simulink model "HvCoorn"  (R2022b)
settings: configuration reference "Icar05FusaMdlCfg" (kept outside this file)
undefined symbols (not defined in the file): BMSActSt_ACChrg, BMSActSt_DCChrg, BMSActSt_disconnect, BMSActSt_offline, BMSActSt_online, BMSActSt_undefined, BMSMainNegRlySt_Clsd_SC, BMSMainNegRlySt_Open_SC, BMSMainNegRlySt_StuckInClsd_SC, BMSMainNegRlySt_StuckInOpen_SC, BMSMainPosRlySt_Clsd_SC, BMSMainPosRlySt_Open_SC, BMSMainPosRlySt_StuckInClsd_SC, BMSPrecRlySt_StuckInOpen_SC, BMSReqSt_ACChrg, BMSReqSt_DCChrg, BMSReqSt_emergencyOffline, BMSReqSt_offline, BMSReqSt_online, Chrg_stCycleBookMod_SC, Chrg_stSingleBookMod_SC, CmpgMod_stInactv_SC, DCDCActSt_buck, DCDCActSt_connected, DCDCActSt_disconnected, DCDCReqSt_buck, DCDCReqSt_standby, EngStrtStop_RefuModDft_SC, EPBActSt_Appld_SC, GearLvr_stDrvGearD_SC, GearLvr_stDrvGearN_SC, GearLvr_stDrvGearP_SC, GearLvr_stDrvGearR_SC, hpp_bACChargeLinkIni_C, hpp_bACChargeLinkOKIni_C, hpp_bAcChgEnaIni_C, hpp_bAcChgPauseIni_C, hpp_bAcLinkTempErrIni_C, hpp_bBattWarmReqIni_C, hpp_bHvilHwErrIni_C, hpp_bHvilStOkIni_C, hpp_bHvRelayClsActIni_C, hpp_bHvRelayOpnActIni_C, hpp_bHvRelayStuckIni_C, hpp_bParked4ChDchgIni_C, hpp_bRemLvBatMntnReqIni_C, hpp_bStartUpReqIni_C, hpp_stHvilCanIni_C, hpp_stWarmTimeCfgRespIni_C, HvCoorn_bAuthEnaSwt_C, HvCoorn_bAuthFailSpdLimOvrd_C, HvCoorn_bAuthFailSpdLimOvrdVal_C, HvCoorn_bAuthStrt_C, HvCoorn_bBMSUnexpdDcnctFailEna_C, HvCoorn_bBuck2RdyBypDCDCEna_C, HvCoorn_bDCChrgFctCfg_C, HvCoorn_bDcChrgWkupEnaChrgLink_C, HvCoorn_bDCDcnct4ACEna_C, HvCoorn_bDCNotBuck2ShtdwnEna_C, HvCoorn_bDrvrLevNotRdyEna_C ... (+295)
libraries: ITKLib x213, simulink x61
(part 9 of 12)

== system HvCoorn/HvCoorn/HVP_HighVoltagePowerOnOffProcedure/A01_HighvoltPowerUpReq/B01_HvRelayClsAct ==
  note: This subsystem calculates the actual status of Hv relay, for example closed, open, stuck, based on the actual status of Hv battery, the main positive relay, the main negative relay, and the precharge relay.
  note: Documentation
  icbms_stMainPosRly : Inport
  icbms_stPrecRly : Inport  Port=2
  icbms_stMainNegRly : Inport  Port=3
  icbms_stHvBat : Inport  Port=4
  Copyright : simulink/Model-Wide Utilities/Model Info  Frame=on  DisplayStringWithTags=|  HorizontalTextAlignment=Left  LeftAlignmentValue=0.02
      | © ITK Engineering Technology (Wu Xi) Co., Ltd. (ITKC)
      | 
      | Model Version: %<ModelVersion>
      | Date: %<LastModificationDate>
  InlineDescription : ITKLib/Special/InlineDescription  Tag=HideFromReport  Description=高压继电器状态确认  ShowInLibBrowser=0  RefreshPar=0
      settings: SourceProductName=ITKC_Lib
  Logical Operator1 : Logic  Operator=OR  Inputs=3  AllPortsSameDT=off  OutDataTypeStr=boolean
  Logical Operator2 : Logic  Operator=OR  Inputs=3  AllPortsSameDT=off  OutDataTypeStr=boolean
  Logical Operator3 : Logic  Operator=OR  AllPortsSameDT=off  OutDataTypeStr=boolean
  Logical Operator4 : Logic  AllPortsSameDT=off  OutDataTypeStr=boolean
  Logical Operator5 : Logic  Operator=OR  AllPortsSameDT=off  OutDataTypeStr=boolean
  Logical Operator6 : Logic  AllPortsSameDT=off  OutDataTypeStr=boolean
  Logical Operator7 : Logic  Operator=OR  AllPortsSameDT=off  OutDataTypeStr=boolean
  Relational Operator{1..13} (13 alike) : RelationalOperator  Operator===  OutDataTypeStr=boolean  InputSameDT=off
  Switch : Switch  Criteria=u2 ~= 0  SaturateOnIntegerOverflow=off  InputSameDT=off
      settings: AttributesFormatString=Criteria : %<Criteria>
  Unit detailed design : simulink/Model-Wide Utilities/DocBlock  Tag=HideFromReport  DocumentType=Text
      content=|
      | SMiVCU-3250 - 高压继电器闭合标志位
      | <电池状态>为0x4:online，或0x9：ACChrg，或0x8：DCChrg，则认为当前高压继电器为闭合状态，激活[高压继电器闭合标志位]。
      |
      | SMiVCU-3251 - 高压继电器断开标志位
      | <电池状态>为0x1：offline，或0x0：undefined，或<主正继电器状态>为0x1：open，或<主负继电器状态>为0x1：open，则认为当前高压继电器为断开状态，激活[高压继电器断开标志位]。
      |
      | SMiVCU-3252 - 高压继电器粘连标志位
      | 同时满足以下条件，则激活[高压继电器粘连标志位]
      | 1.<主正继电器状态>为0x4：StucInClsd或<预充继电器状态>为0x3：StucInOpen；
      | 2.<主负继电器状态>为0x4：StucInClsd或0x3：StucInOpen；
  hpp_tiHvilOkDelay_C : Constant  Description=[0]  Value=HvCoorn_bHvRlyClsJudgByMod_C
      settings: AttributesFormatString=%<Description>
  icbms_acCharge : Constant  Description=[9]  Value=BMSActSt_ACChrg  OutDataTypeStr=uint8
      settings: AttributesFormatString=[9]
  icbms_dcCharge : Constant  Description=[8]  Value=BMSActSt_DCChrg  OutDataTypeStr=uint8
      settings: AttributesFormatString=[8]
  icbms_offline : Constant  Description=[1]  Value=BMSActSt_offline  OutDataTypeStr=uint8
      settings: AttributesFormatString=[1]
  icbms_online : Constant  Description=[4]  Value=BMSActSt_online  OutDataTypeStr=uint8
      settings: AttributesFormatString=[4]
  icbms_undefined : Constant  Description=[0]  Value=BMSActSt_undefined  OutDataTypeStr=uint8
      settings: AttributesFormatString=[0]
  icbms_undefined1 : Constant  Description=[4]  Value=BMSMainPosRlySt_StuckInClsd_SC  OutDataTypeStr=uint8
      settings: AttributesFormatString=%<Description>
  icbms_undefined2 : Constant  Description=[4]  Value=BMSMainNegRlySt_StuckInClsd_SC  OutDataTypeStr=uint8
      settings: AttributesFormatString=%<Description>
  icbms_undefined3 : Constant  Description=[3]  Value=BMSMainNegRlySt_StuckInOpen_SC  OutDataTypeStr=uint8
      settings: AttributesFormatString=%<Description>
  icbms_undefined4 : Constant  Description=[3]  Value=BMSPrecRlySt_StuckInOpen_SC  OutDataTypeStr=uint8
      settings: AttributesFormatString=%<Description>
  icbms_undefined5 : Constant  Description=[2]  Value=BMSMainNegRlySt_Clsd_SC  OutDataTypeStr=uint8
      settings: AttributesFormatString=%<Description>
  icbms_undefined6 : Constant  Description=[2]  Value=BMSMainPosRlySt_Clsd_SC  OutDataTypeStr=uint8
      settings: AttributesFormatString=%<Description>
  icbms_undefined7 : Constant  Description=[1]  Value=BMSMainNegRlySt_Open_SC  OutDataTypeStr=uint8
      settings: AttributesFormatString=%<Description>
  icbms_undefined8 : Constant  Description=[1]  Value=BMSMainPosRlySt_Open_SC  OutDataTypeStr=uint8
      settings: AttributesFormatString=%<Description>
  HvCoorn_bHvRlyClsAct : Outport  VectorParamsAs1DForOutWhenUnconnected=off
  HvCoorn_bHvRlyOpenAct : Outport  Port=2  VectorParamsAs1DForOutWhenUnconnected=off
  HvCoorn_bHvRlyStuck : Outport  Port=3  VectorParamsAs1DForOutWhenUnconnected=off
  wires:
  icbms_stMainPosRly/1 -> [icbms_stMainPosRly], Relational Operator8/1
  icbms_undefined1/1 -> Relational Operator8/2
  Relational Operator8/1 -> Logical Operator3/1
  icbms_stPrecRly/1 -> Relational Operator9/1
  icbms_stMainNegRly/1 -> [icbms_stMainNegRly], Relational Operator6/1, Relational Operator10/1
  Relational Operator9/1 -> Logical Operator3/2
  Logical Operator3/1 -> Logical Operator4/1
  Relational Operator10/1 -> Logical Operator5/1
  Logical Operator4/1 -> HvCoorn_bHvRlyStuck/1
  icbms_stHvBat/1 -> Relational Operator5/1, Relational Operator1/1, Relational Operator4/1, Relational Operator3/1, Relational Operator2/1
  icbms_acCharge/1 -> Relational Operator3/2
  icbms_dcCharge/1 -> Relational Operator4/2
  Relational Operator3/1 -> Logical Operator1/2
  Relational Operator4/1 -> Logical Operator1/3
  icbms_offline/1 -> Relational Operator1/2
  Relational Operator1/1 -> Logical Operator2/2
  Relational Operator5/1 -> Logical Operator2/3
  icbms_online/1 -> Relational Operator2/2
  Relational Operator2/1 -> Logical Operator1/1
  Logical Operator2/1 -> HvCoorn_bHvRlyOpenAct/1
  Switch/1 -> HvCoorn_bHvRlyClsAct/1
  icbms_undefined/1 -> Relational Operator5/2
  icbms_undefined2/1 -> Relational Operator10/2
  Relational Operator6/1 -> Logical Operator5/2
  icbms_undefined3/1 -> Relational Operator6/2
  icbms_undefined4/1 -> Relational Operator9/2
  Logical Operator5/1 -> Logical Operator4/2
  [icbms_stMainNegRly] -> Relational Operator13/1
  icbms_undefined8/1 -> Relational Operator12/2
  [icbms_stMainPosRly] -> Relational Operator12/1
  icbms_undefined7/1 -> Relational Operator13/2
  Relational Operator12/1 -> Logical Operator7/1
  Relational Operator13/1 -> Logical Operator7/2
  Logical Operator7/1 -> Logical Operator2/1
  [icbms_stMainNegRly] -> Relational Operator7/1
  Relational Operator11/1 -> Logical Operator6/1
  Relational Operator7/1 -> Logical Operator6/2
  icbms_undefined6/1 -> Relational Operator11/2
  icbms_undefined5/1 -> Relational Operator7/2
  [icbms_stMainPosRly] -> Relational Operator11/1
  Logical Operator1/1 -> Switch/1
  hpp_tiHvilOkDelay_C/1 -> Switch/2
  Logical Operator6/1 -> Switch/3

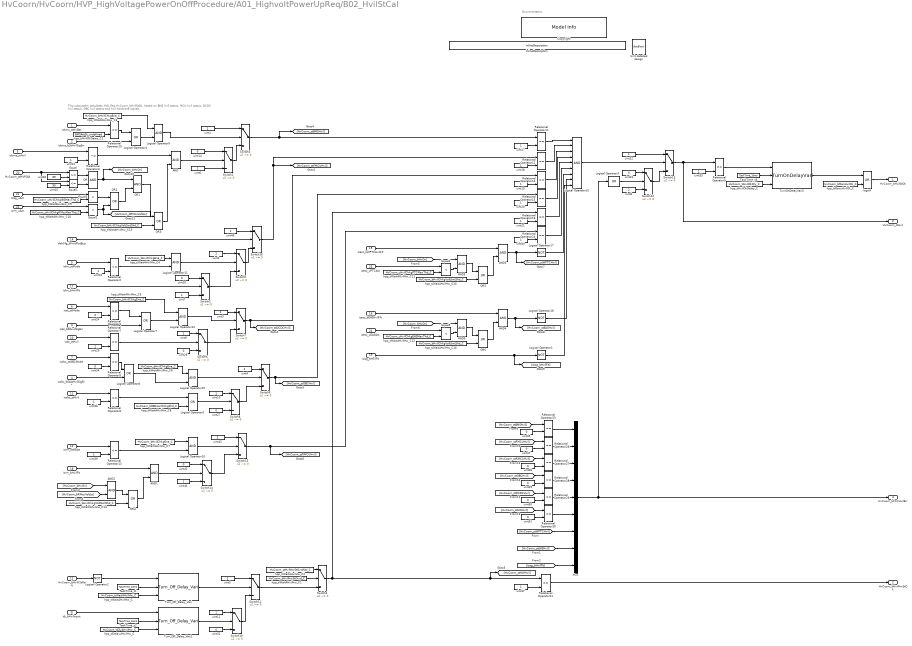
== system HvCoorn/HvCoorn/HVP_HighVoltagePowerOnOffProcedure/A01_HighvoltPowerUpReq/B02_HvilStCal ==
  note: This subsystem calculates HVIL flag HvCoorn_bHvilStOk, based on BMS hvil status, MCU hvil status, DCDC hvil status, OBC hvil status and hvil hardware signals .
  note: Documentation
  icbms_stHvBat : Inport
  icbms_bStHvilSigErr : Inport  Port=2
  icdc_bStHvilSigErr : Inport  Port=3
  icobc_bStAcHvilSigErr : Inport  Port=4
  icfm_stMode : Inport  Port=5
  icdc_stMode : Inport  Port=6
  icobc_stOBCMode : Inport  Port=7
  idi_bHvilInput : Inport  Port=8
  icbms_stHvil : Inport  Port=9
  icdc_stHvil : Inport  Port=10
  icobc_stHvil : Inport  Port=11
  HvCoorn_bHvilClsReq : Inport  Port=12
  icrm_stMode : Inport  Port=13
  VehCfg_bFrntMotByp : Inport  Port=14
  icecc_bWPTCHvilFlt : Inport  Port=15
  icecc_bEASHvilFlt : Inport  Port=16
  icfm_bHvilFlt : Inport  Port=17
  icrm_bHvilFlt : Inport  Port=18
  icisg_bHvilFlt : Inport  Port=19
  HvCoorn_stHVPOld : Inport  Port=20
  icisg_uAct : Inport  Port=21
  icrm_uAct : Inport  Port=22
  icecc_uPTCAct : Inport  Port=23
  icecc_uEASAct : Inport  Port=24
  AND{,1..6} (7 alike) : Logic  OutDataTypeStr=boolean
  Copyright : simulink/Model-Wide Utilities/Model Info  Frame=on  DisplayStringWithTags=|  HorizontalTextAlignment=Left  LeftAlignmentValue=0.02
      | © ITK Engineering Technology (Wu Xi) Co., Ltd. (ITKC)
      | 
      | Model Version: %<ModelVersion>
      | Date: %<LastModificationDate>
  Equal : RelationalOperator  OutDataTypeStr=boolean  RndMeth=Simplest  InputSameDT=off
  Equal1 : RelationalOperator  Operator=<=  OutDataTypeStr=boolean  RndMeth=Simplest  InputSameDT=off
  Equal{2..5} (4 alike) : RelationalOperator  Operator=<  OutDataTypeStr=boolean
  InlineDescription : ITKLib/Special/InlineDescription  Tag=HideFromReport  Description=互锁状态确认  ShowInLibBrowser=0  RefreshPar=0
      settings: SourceProductName=ITKC_Lib
  Logical Operator{1..2,17..18} (4 alike) : Logic  Operator=NOT  Inputs=1  AllPortsSameDT=off  OutDataTypeStr=boolean
  Logical Operator10 : Logic  Inputs=9  AllPortsSameDT=off  OutDataTypeStr=boolean
  Logical Operator{9,11..12,15..16} (5 alike) : Logic  AllPortsSameDT=off  OutDataTypeStr=boolean
  Logical Operator3 : Logic  Operator=OR  Inputs=1  AllPortsSameDT=off  OutDataTypeStr=boolean
  Logical Operator{4..5,7..8} (4 alike) : Logic  Operator=OR  AllPortsSameDT=off  OutDataTypeStr=boolean
  Mux : Mux  Inputs=9
  OR : Logic  OutDataTypeStr=boolean
  OR1 : Logic  OutDataTypeStr=boolean
  OR{2..6} (5 alike) : Logic  Operator=OR  OutDataTypeStr=boolean
  Relational Operator{4..5,7..12,14..16,21,23..24,26..30} (19 alike) : RelationalOperator  Operator===  OutDataTypeStr=boolean  InputSameDT=off
  Relational Operator13 : RelationalOperator  Operator=<=  OutDataTypeStr=boolean  InputSameDT=off
  Relational Operator2 : RelationalOperator  Operator=<=  OutDataTypeStr=boolean  InputSameDT=off
  Relational Operator3 : RelationalOperator  Operator=~=  OutDataTypeStr=boolean  InputSameDT=off
  Switch{1..16} (16 alike) : Switch  Criteria=u2 ~= 0  OutDataTypeStr=uint8  SaturateOnIntegerOverflow=off  InputSameDT=off
  TaskTime_s1 : Constant  Value=TaskTime_10ms
      settings: AttributesFormatString=[0.01]
  TaskTime_s2 : Constant  Value=TaskTime_10ms
      settings: AttributesFormatString=[0.01]
  TaskTime_s5 : Constant  Value=TaskTime_10ms
      settings: AttributesFormatString=[0.01]
  TurnOnDelayVari3 : ITKLib/TimeCounter/TurnOnDelayVari
      settings: AttributesFormatString=TurnOnDelay  SourceProductName=ITKC_Lib
  Turn_Off_Delay_Vari : ITKLib/TimeCounter/Turn_Off_Delay_Vari
      settings: AttributesFormatString=TurnOffDelay  SourceProductName=ITKC_Lib
  Turn_Off_Delay_Vari1 : ITKLib/TimeCounter/Turn_Off_Delay_Vari
      settings: AttributesFormatString=TurnOffDelay  SourceProductName=ITKC_Lib
  Unit detailed design : simulink/Model-Wide Utilities/DocBlock  Tag=HideFromReport  DocumentType=Text
      content=|
      | SMiVCU-3254 - 高压互锁状态
      | 以下条件同时满足，则[高压互锁状态]为0x1：OK，否则为0x0：Not OK：
      | 1.<动力电池包高压互锁状态>为0x1：Connected；
      | 2.<充电机高压互锁状态>为0x1：Connected或<OBC充电连接状态>为0x0：Disconnected。
      |
      | SMiVCU-3255 - 高压互锁OK标志位
      | [高压互锁状态]为0x1：OK，并持续一定时间（HvCoorn_tiHvilOkDly_C，初始值0.03）后激活[高压互锁OK标志位]。
  hpp_bManuHvilOk_C : Constant  Description=[0]  Value=HvCoorn_bManHvilOk_C  OutDataTypeStr=boolean
      settings: AttributesFormatString=%<Description>
  hpp_tiDelay4HvilHw_C : Constant  Description=[0.1]  Value=HvCoorn_tiDly4HvilHw_C
      settings: AttributesFormatString=%<Description>
  hpp_tiHvilOkDelay_C : Constant  Description=[0.03]  Value=HvCoorn_tiHvilOkDly_C
      settings: AttributesFormatString=%<Description>
  hpp_tiHvilOkDelay_C1 : Constant  Description=[0]  Value=BMSActSt_undefined
      settings: AttributesFormatString=[0]
  hpp_tiWait4HvilHw_C : Constant  Description=[0.08]  Value=HvCoorn_tiWait4HvilHw_C
      settings: AttributesFormatString=%<Description>
  hpp_tiWait4HvilHw_C1 : Constant  Description=[1]  Value=HvCoorn_bHvilHwStOvrd_C
      settings: AttributesFormatString=%<Description>
  hpp_tiWait4HvilHw_C10 : Constant  Description=[200]  Value=HvCoorn_uHvilChkgRMcuMaxThd_C
      settings: AttributesFormatString=%<Description>
  hpp_tiWait4HvilHw_C11 : Constant  Description=[200]  Value=HvCoorn_uHvilChkgPTCMaxThd_C
      settings: AttributesFormatString=%<Description>
  hpp_tiWait4HvilHw_C12 : Constant  Description=[200]  Value=HvCoorn_uHvilChkgEASMaxThd_C
      settings: AttributesFormatString=%<Description>
  hpp_tiWait4HvilHw_C{13..16} (4 alike) : Constant  Description=[1]  Value=HvCoorn_bHvilChkgVoltSwtShd_C
      settings: AttributesFormatString=%<Description>
  hpp_tiWait4HvilHw_C2 : Constant  Description=[1]  Value=HvCoorn_stHvilHwStOvrdVal_C
      settings: AttributesFormatString=%<Description>
  hpp_tiWait4HvilHw_C{3..7} (5 alike) : Constant  Description=[0]  Value=HvCoorn_bHvilChkgEna_C
      settings: AttributesFormatString=%<Description>
  hpp_tiWait4HvilHw_C8 : Constant  Description=[1]  Value=HvCoorn_bOBCHvilChkgShd_C
      settings: AttributesFormatString=%<Description>
  hpp_tiWait4HvilHw_C9 : Constant  Description=[200]  Value=HvCoorn_uHvilChkgISGMaxThd_C
      settings: AttributesFormatString=%<Description>
  logic4 : Logic  Operator=OR  AllPortsSameDT=off  OutDataTypeStr=boolean
  uint{1..5,8,43} (7 alike) : Constant  Description=Checking  Value=2  OutDataTypeStr=uint8
      settings: AttributesFormatString=|
      | %<OutDataTypeStr>
      | %<Description>
  uint{6..7,9..11,17..22,33,37,40,44,46} (16 alike) : Constant  Description=Ok  OutDataTypeStr=uint8
      settings: AttributesFormatString=|
      | %<OutDataTypeStr>
      | %<Description>
  uint12 : Constant  Description=BMSClosed  OutDataTypeStr=uint8
      settings: AttributesFormatString=|
      | %<OutDataTypeStr>
      | %<Description>
  uint13 : Constant  Description=MCUInitial  OutDataTypeStr=uint8
      settings: AttributesFormatString=|
      | %<OutDataTypeStr>
      | %<Description>
  uint{14,16,23,26..27,32,35,42,47..51} (13 alike) : Constant  Description=NotOk  Value=0  OutDataTypeStr=uint8
      settings: AttributesFormatString=|
      | %<OutDataTypeStr>
      | %<Description>
  uint15 : Constant  Value=95  OutDataTypeStr=uint8  SampleTime=-1
      settings: AttributesFormatString=%<OutDataTypeStr>
  uint24 : Constant  Description=DCDCInitial  Value=0  OutDataTypeStr=uint8
      settings: AttributesFormatString=|
      | %<OutDataTypeStr>
      | %<Description>
  uint25 : Constant  Description=DCDCClosed  OutDataTypeStr=uint8
      settings: AttributesFormatString=|
      | %<OutDataTypeStr>
      | %<Description>
  uint28 : Constant  Value=89  OutDataTypeStr=uint8  SampleTime=-1
      settings: AttributesFormatString=%<OutDataTypeStr>
  uint34 : Constant  Description=OBCInitial  Value=0  OutDataTypeStr=uint8
      settings: AttributesFormatString=|
      | %<OutDataTypeStr>
      | %<Description>
  uint36 : Constant  Description=OBCClosed  OutDataTypeStr=uint8
      settings: AttributesFormatString=|
      | %<OutDataTypeStr>
      | %<Description>
  uint39 : Constant  Description=MCUInitial  OutDataTypeStr=uint8
      settings: AttributesFormatString=|
      | %<OutDataTypeStr>
      | %<Description>
  HvCoorn_bHvilStOk : Outport  VectorParamsAs1DForOutWhenUnconnected=off
  HvCoorn_bHvilHwStOk : Outport  Port=2  VectorParamsAs1DForOutWhenUnconnected=off
  HvCoorn_stHvil : Outport  Port=3  VectorParamsAs1DForOutWhenUnconnected=off
  HvCoorn_bCtrlrHvilErr : Outport  Port=4  VectorParamsAs1DForOutWhenUnconnected=off
  wires:
  icbms_stHvil/1 -> Relational Operator3/1
  uint22/1 -> Switch13/1
  icbms_stHvBat/1 -> Relational Operator10/1
  icfm_stMode/1 -> Relational Operator2/1
  uint13/1 -> Relational Operator2/2
  uint24/1 -> Relational Operator4/2
  icdc_stMode/1 -> Relational Operator4/1
  uint34/1 -> Relational Operator5/2
  icobc_stOBCMode/1 -> Relational Operator5/1
  HvCoorn_bHvilClsReq/1 -> Logical Operator2/1
  icdc_stHvil/1 -> Relational Operator7/1
  icobc_stHvil/1 -> Relational Operator8/1
  Switch13/1 -> HvCoorn_stHvil/1, Relational Operator9/1
  hpp_bManuHvilOk_C/1 -> logic4/2
  uint33/1 -> Relational Operator9/2
  logic4/1 -> HvCoorn_bHvilStOk/1
  Relational Operator21/1 -> HvCoorn_bHvilHwStOk/1
  hpp_tiWait4HvilHw_C/1 -> Turn_Off_Delay_Vari/3
  Logical Operator2/1 -> Turn_Off_Delay_Vari/1
  TaskTime_s2/1 -> Turn_Off_Delay_Vari1/2
  hpp_tiDelay4HvilHw_C/1 -> Turn_Off_Delay_Vari1/3
  uint12/1 -> Relational Operator3/2
  Logical Operator9/1 -> Switch3/2
  Switch1/1 -> Switch3/3
  uint25/1 -> Relational Operator7/2
  uint36/1 -> Relational Operator8/2
  Logical Operator11/1 -> Switch5/2
  icfm_bHvilFlt/1 -> Switch2/2
  Switch2/1 -> Switch5/3
  Logical Operator12/1 -> Switch7/2
  Relational Operator7/1 -> Switch6/2
  Switch6/1 -> Switch7/3
  Logical Operator15/1 -> Switch9/2
  Switch8/1 -> Switch9/3
  Turn_Off_Delay_Vari/1 -> Switch11/2
  uint32/1 -> Switch10/3
  Switch10/1 -> Switch11/3
  uint1/1 -> Switch3/1
  Relational Operator11/1 -> Logical Operator10/1
  uint21/1 -> Relational Operator16/2
  Switch3/1 -> Relational Operator11/1, [HvCoorn_stBMSHvil]
  Relational Operator16/1 -> Logical Operator10/5
  Relational Operator15/1 -> Logical Operator10/4
  Relational Operator14/1 -> Logical Operator10/3
  Relational Operator12/1 -> Logical Operator10/2
  Switch16/1 -> Relational Operator12/1, [HvCoorn_stFMCUHvil]
  Switch7/1 -> Relational Operator14/1, [HvCoorn_stDCDCHvil]
  Switch9/1 -> Relational Operator15/1, [HvCoorn_stOBCHvil]
  Switch4/1 -> [HvCoorn_stHWHvil], Relational Operator21/1, Relational Operator16/1
  uint23/1 -> Switch12/1
  Logical Operator10/1 -> Switch13/2
  Switch12/1 -> Switch13/3
  Mux/1 -> Logical Operator3/1, HvCoorn_bCtrlrHvilErr/1
  uint8/1 -> Switch12/3
  Relational Operator9/1 -> TurnOnDelayVari3/1
  hpp_tiHvilOkDelay_C/1 -> TurnOnDelayVari3/3
  TurnOnDelayVari3/1 -> logic4/1
  Relational Operator10/1 -> Logical Operator4/1
  icbms_bStHvilSigErr/1 -> Logical Operator4/2
  Relational Operator4/1 -> Logical Operator7/1
  icdc_bStHvilSigErr/1 -> Logical Operator7/2
  Relational Operator5/1 -> Logical Operator8/1
  icobc_bStAcHvilSigErr/1 -> Logical Operator8/2
  idi_bHvilInput/1 -> Turn_Off_Delay_Vari1/1
  Turn_Off_Delay_Vari1/1 -> Switch10/2
  TaskTime_s5/1 -> TurnOnDelayVari3/2
  hpp_tiHvilOkDelay_C1/1 -> Relational Operator10/2
  uint2/1 -> Switch5/1
  uint3/1 -> Switch7/1
  uint4/1 -> Switch9/1
  uint5/1 -> Switch11/1
  uint9/1 -> Switch6/1
  uint10/1 -> Switch8/1
  uint11/1 -> Switch10/1
  uint17/1 -> Relational Operator11/2
  uint18/1 -> Relational Operator12/2
  uint19/1 -> Relational Operator14/2
  uint20/1 -> Relational Operator15/2
  uint26/1 -> Switch6/3
  uint27/1 -> Switch8/3
  uint37/1 -> Relational Operator21/2
  TaskTime_s1/1 -> Turn_Off_Delay_Vari/2
  hpp_tiWait4HvilHw_C1/1 -> Switch4/2
  Switch11/1 -> Switch4/3
  hpp_tiWait4HvilHw_C2/1 -> Switch4/1
  uint43/1 -> Switch15/1
  Switch14/1 -> Switch15/3
  Logical Operator16/1 -> Switch15/2
  uint39/1 -> Relational Operator13/2
  icrm_stMode/1 -> Relational Operator13/1
  uint40/1 -> Relational Operator24/2
  Relational Operator24/1 -> Logical Operator10/6
  Switch15/1 -> [HvCoorn_stRMCUHvil], Relational Operator24/1
  Switch5/1 -> Switch16/3
  VehCfg_bFrntMotByp/1 -> Switch16/2
  uint46/1 -> Switch16/1
  Logical Operator4/1 -> Logical Operator9/2
  hpp_tiWait4HvilHw_C3/1 -> Logical Operator9/1
  hpp_tiWait4HvilHw_C4/1 -> Logical Operator11/1
  Relational Operator2/1 -> Logical Operator11/2
  hpp_tiWait4HvilHw_C5/1 -> Logical Operator12/1
  Logical Operator7/1 -> Logical Operator12/2
  hpp_tiWait4HvilHw_C6/1 -> Logical Operator15/1
  Logical Operator8/1 -> Logical Operator15/2
  hpp_tiWait4HvilHw_C7/1 -> Logical Operator16/1
  Relational Operator13/1 -> Logical Operator16/2
  AND3/1 -> Logical Operator17/1, [HvCoorn_stWPTCHvil]
  Logical Operator17/1 -> Logical Operator10/7
  AND4/1 -> Logical Operator18/1, [HvCoorn_stEASHvil]
  Logical Operator18/1 -> Logical Operator10/8
  uint35/1 -> Relational Operator23/2
  [HvCoorn_stBMSHvil] -> Relational Operator23/1
  uint47/1 -> Relational Operator26/2
  [HvCoorn_stFMCUHvil] -> Relational Operator26/1
  uint48/1 -> Relational Operator27/2
  [HvCoorn_stRMCUHvil] -> Relational Operator27/1
  uint49/1 -> Relational Operator28/2
  [HvCoorn_stOBCHvil] -> Relational Operator28/1
  [HvCoorn_stDCDCHvil] -> Relational Operator29/1
  uint50/1 -> Relational Operator29/2
  uint51/1 -> Relational Operator30/2
  [HvCoorn_stHWHvil] -> Relational Operator30/1
  Relational Operator23/1 -> Mux/1
  [HvCoorn_stEASHvil] -> Mux/8
  Relational Operator26/1 -> Mux/2
  Relational Operator27/1 -> Mux/3
  Relational Operator28/1 -> Mux/4
  Relational Operator29/1 -> Mux/5
  Relational Operator30/1 -> Mux/6
  [HvCoorn_stWPTCHvil] -> Mux/7
  Logical Operator3/1 -> Switch12/2
  uint16/1 -> Switch2/1
  uint7/1 -> Switch2/3
  uint42/1 -> Switch14/1
  uint44/1 -> Switch14/3
  icisg_bHvilFlt/1 -> Logical Operator1/1, [icisg_bHvilFlt]
  Logical Operator1/1 -> Logical Operator10/9
  [icisg_bHvilFlt] -> Mux/9
  Relational Operator8/1 -> Logical Operator5/1
  Logical Operator5/1 -> Switch8/2
  hpp_tiWait4HvilHw_C8/1 -> Logical Operator5/2
  Equal1/1 -> OR/2
  uint15/1 -> Equal1/2
  uint28/1 -> Equal/2
  Equal/1 -> OR/1
  HvCoorn_stHVPOld/1 -> Equal/1, Equal1/1
  icisg_uAct/1 -> Equal3/1
  hpp_tiWait4HvilHw_C9/1 -> Equal3/2
  OR/1 -> [HvCoorn_bHvOn], OR1/1
  uint14/1 -> Switch1/1
  uint6/1 -> Switch1/3
  AND/1 -> Switch1/2
  Relational Operator3/1 -> AND/1
  hpp_tiWait4HvilHw_C10/1 -> Equal2/2
  icrm_uAct/1 -> Equal2/1
  Equal3/1 -> OR2/1
  Equal2/1 -> OR2/2, [HvCoorn_bRMcuVoltLo]
  OR2/1 -> OR1/2
  AND1/1 -> Switch14/2
  icrm_bHvilFlt/1 -> AND1/1
  [HvCoorn_bRMcuVoltLo] -> AND2/2
  [HvCoorn_bHvOn] -> AND2/1
  icecc_bWPTCHvilFlt/1 -> AND3/1
  hpp_tiWait4HvilHw_C11/1 -> Equal4/2
  icecc_uPTCAct/1 -> Equal4/1
  Equal4/1 -> AND5/2
  icecc_uEASAct/1 -> Equal5/1
  hpp_tiWait4HvilHw_C12/1 -> Equal5/2
  icecc_bEASHvilFlt/1 -> AND4/1
  OR1/1 -> OR3/1
  OR3/1 -> AND/2
  hpp_tiWait4HvilHw_C13/1 -> OR3/2
  hpp_tiWait4HvilHw_C14/1 -> OR4/2
  AND2/1 -> OR4/1
  OR4/1 -> AND1/2
  hpp_tiWait4HvilHw_C15/1 -> OR5/2
  [HvCoorn_bHvOn] -> AND5/1
  AND5/1 -> OR5/1
  OR5/1 -> AND3/2
  Equal5/1 -> AND6/2
  [HvCoorn_bHvOn] -> AND6/1
  hpp_tiWait4HvilHw_C16/1 -> OR6/2
  AND6/1 -> OR6/1
  OR6/1 -> AND4/2

== system HvCoorn/HvCoorn/HVP_HighVoltagePowerOnOffProcedure/A01_HighvoltPowerUpReq/B03_ChgrPortOverTemp ==
  note: This subsystem calculates AC Charger over temperature flag based on L1 temperature and N temperature, also calculates DC Charger over temperature flag based on charger temperature.
  note: Documentation
  ian_tAcChrgrL1Temp : Inport
  ian_tAcChrgrNTemp : Inport  Port=2
  HvCoorn_bACChrgLink : Inport  Port=3
  ian_tDcChrgrTemp1 : Inport  Port=4
  ian_tDcChrgrTemp2 : Inport  Port=5
  HvCoorn_bDCChargeLink : Inport  Port=6
  Copyright : simulink/Model-Wide Utilities/Model Info  Frame=on  DisplayStringWithTags=|  HorizontalTextAlignment=Left  LeftAlignmentValue=0.02
      | © ITK Engineering Technology (Wu Xi) Co., Ltd. (ITKC)
      | 
      | Model Version: %<ModelVersion>
      | Date: %<LastModificationDate>
  GreaterOrEqual : RelationalOperator  OutDataTypeStr=boolean
  GreaterOrEqual1 : RelationalOperator  OutDataTypeStr=boolean
  HysteresisA : ITKLib/Hysteresis/HysteresisA  Description=HysteresisA
      settings: AttributesFormatString=%<Description>  SourceProductName=ITKC_Lib
  HysteresisA1 : ITKLib/Hysteresis/HysteresisA  Description=HysteresisA
      settings: AttributesFormatString=%<Description>  SourceProductName=ITKC_Lib
  InlineDescription : ITKLib/Special/InlineDescription  Tag=HideFromReport  Description=充电连接温度故障  ShowInLibBrowser=0  RefreshPar=0
      settings: SourceProductName=ITKC_Lib
  Logical Operator1 : Logic  Operator=NOT  Inputs=1  AllPortsSameDT=off  OutDataTypeStr=boolean
  Logical Operator3 : Logic  Operator=NOT  Inputs=1  AllPortsSameDT=off  OutDataTypeStr=boolean
  Logical Operator5 : Logic  Operator=OR  AllPortsSameDT=off  OutDataTypeStr=boolean
  Logical Operator59 : Logic  Operator=OR  AllPortsSameDT=off  OutDataTypeStr=boolean
  Logical Operator6 : Logic  Operator=OR  Inputs=1  AllPortsSameDT=off  OutDataTypeStr=boolean
  Logical Operator60 : Logic  Operator=OR  Inputs=1  AllPortsSameDT=off  OutDataTypeStr=boolean
  Mux : Mux  Inputs=2
  Mux1 : Mux  Inputs=2
  Sum1 : Sum  Inputs=+-  SaturateOnIntegerOverflow=on
  Sum3 : Sum  Inputs=+-  SaturateOnIntegerOverflow=on
  Switch1 : Switch  Criteria=u2 ~= 0  SaturateOnIntegerOverflow=off  InputSameDT=off
  Switch2 : Switch  Criteria=u2 ~= 0  SaturateOnIntegerOverflow=off  InputSameDT=off
  TaskTime_s{1..4} (4 alike) : Constant  Value=TaskTime_10ms
      settings: AttributesFormatString=[0.01]
  TurnOnDelayVari{,1..3} (4 alike) : ITKLib/TimeCounter/TurnOnDelayVari
      settings: AttributesFormatString=TurnOnDelay  SourceProductName=ITKC_Lib
  Unit Delay1 : UnitDelay  SampleTime=-1  HasFrameUpgradeWarning=on
      settings: AttributesFormatString=<initial=%<X0>>
  Unit Delay3 : UnitDelay  SampleTime=-1  HasFrameUpgradeWarning=on
      settings: AttributesFormatString=<initial=%<X0>>
  Unit detailed design : simulink/Model-Wide Utilities/DocBlock  Tag=HideFromReport  DocumentType=Text
      content=|
      | SMiVCU-3263 - DC充电连接温度故障标志位
      | 若<DC充电口温度1>或<DC充电口温度2>大于一定值（HvCoorn_tDcLinkTempErr_C，初始值100℃），或[DC充电连接标志位]激活后单个周期的变化值大于一定值（HvCoorn_tDcLinkTempIncErr_C，初始值50℃），TurnOnDelay一定时间（HvCoorn_tiChgLinkOverTempDeb_C，初始值0.03s）后激活[DC充电连接温度故障标志位]。
  hpp_tAcLinkTempErrHi_C : Constant  Description=[5000]  Value=HvCoorn_tAcLinkTempErrHi_C
      settings: AttributesFormatString=%<Description>
  hpp_tAcLinkTempErrLo_C : Constant  Description=[4950]  Value=HvCoorn_tAcLinkTempErrLo_C
      settings: AttributesFormatString=%<Description>
  hpp_tAcLinkTepmIncErrHi_C : Constant  Description=[5000]  Value=HvCoorn_tAcLinkTepmIncErrHi_C
      settings: AttributesFormatString=%<Description>
  hpp_tAcLinkTepmIncErrLo_C : Constant  Description=[4950]  Value=HvCoorn_tAcLinkTepmIncErrLo_C
      settings: AttributesFormatString=%<Description>
  hpp_tAcLinkTepmIncErrLo_C1 : Constant  Description=[5000]  Value=HvCoorn_tDcLinkTempErr_C
      settings: AttributesFormatString=%<Description>
  hpp_tAcLinkTepmIncErrLo_C2 : Constant  Description=[5000]  Value=HvCoorn_tDcLinkTempIncErr_C
      settings: AttributesFormatString=%<Description>
  hpp_tiChgLinkOverTempDeb_C : Constant  Description=[10000]  Value=HvCoorn_tiChgLinkOverTempDeb_C
      settings: AttributesFormatString=%<Description>
  hpp_tiChgLinkOverTempDeb_C1 : Constant  Description=[10000]  Value=HvCoorn_tiChgLinkOverTempDeb_C
      settings: AttributesFormatString=%<Description>
  hpp_tiLoadAcLinkTemp_C : Constant  Description=[0.1]  Value=HvCoorn_tiLoadAcLinkTemp_C
      settings: AttributesFormatString=%<Description>
  hpp_tiLoadAcLinkTemp_C1 : Constant  Description=[0.1]  Value=HvCoorn_tiLoadDcLinkTemp_C
      settings: AttributesFormatString=%<Description>
  HvCoorn_bACLinkTempErr : Outport  VectorParamsAs1DForOutWhenUnconnected=off
  HvCoorn_bDCLinkTempErr : Outport  Port=2  VectorParamsAs1DForOutWhenUnconnected=off
  wires:
  TurnOnDelayVari1/1 -> HvCoorn_bACLinkTempErr/1
  Logical Operator60/1 -> TurnOnDelayVari1/1
  Switch2/1 -> Unit Delay3/1, Sum1/2  "tLoadInitAcTemp"
  HvCoorn_bACChrgLink/1 -> TurnOnDelayVari/1
  ian_tAcChrgrL1Temp/1 -> Mux/1
  hpp_tiLoadAcLinkTemp_C/1 -> TurnOnDelayVari/3
  Unit Delay3/1 -> Switch2/3
  Logical Operator59/1 -> Logical Operator60/1
  ian_tAcChrgrNTemp/1 -> Mux/2
  TurnOnDelayVari/1 -> Logical Operator1/1
  TaskTime_s2/1 -> TurnOnDelayVari/2
  Logical Operator1/1 -> Switch2/2
  Mux/1 -> HysteresisA/2, Sum1/1, Switch2/1
  Sum1/1 -> HysteresisA1/2
  hpp_tAcLinkTempErrHi_C/1 -> HysteresisA/1
  hpp_tAcLinkTempErrLo_C/1 -> HysteresisA/3
  hpp_tAcLinkTepmIncErrHi_C/1 -> HysteresisA1/1
  hpp_tAcLinkTepmIncErrLo_C/1 -> HysteresisA1/3
  HysteresisA/1 -> Logical Operator59/1
  HysteresisA1/1 -> Logical Operator59/2
  TaskTime_s1/1 -> TurnOnDelayVari1/2
  hpp_tiChgLinkOverTempDeb_C/1 -> TurnOnDelayVari1/3
  TurnOnDelayVari2/1 -> HvCoorn_bDCLinkTempErr/1
  Mux1/1 -> Switch1/1, GreaterOrEqual/1, Sum3/1
  Logical Operator6/1 -> TurnOnDelayVari2/1
  GreaterOrEqual1/1 -> Logical Operator5/2
  hpp_tAcLinkTepmIncErrLo_C2/1 -> GreaterOrEqual1/2
  GreaterOrEqual/1 -> Logical Operator5/1
  Unit Delay1/1 -> Switch1/3
  ian_tDcChrgrTemp1/1 -> Mux1/1
  HvCoorn_bDCChargeLink/1 -> TurnOnDelayVari3/1
  hpp_tAcLinkTepmIncErrLo_C1/1 -> GreaterOrEqual/2
  Sum3/1 -> GreaterOrEqual1/1
  ian_tDcChrgrTemp2/1 -> Mux1/2
  Logical Operator3/1 -> Switch1/2
  TurnOnDelayVari3/1 -> Logical Operator3/1
  Switch1/1 -> Sum3/2, Unit Delay1/1  "tLoadInitDcTemp"
  TaskTime_s3/1 -> TurnOnDelayVari2/2
  hpp_tiChgLinkOverTempDeb_C1/1 -> TurnOnDelayVari2/3
  Logical Operator5/1 -> Logical Operator6/1
  TaskTime_s4/1 -> TurnOnDelayVari3/2
  hpp_tiLoadAcLinkTemp_C1/1 -> TurnOnDelayVari3/3

== system HvCoorn/HvCoorn/HVP_HighVoltagePowerOnOffProcedure/A01_HighvoltPowerUpReq/B04_ParkCheck ==
  note: This subsystem calculates the allowed flag of park charge or discharge based on drive gear P or EPB actual applied status.
  note: Documentation
  HvCoorn_bDCChrgLink : Inport
  idi_bKeyOn : Inport  Port=2
  GearLvr_stDrvGear : Inport  Port=3
  HvCoorn_bACChrgLink : Inport  Port=4
  icepb_stEpbSys : Inport  Port=5
  VehSpd_vVeh : Inport  Port=6
  icobc_bDchrgrCnct : Inport  Port=7
  AND : Logic  OutDataTypeStr=boolean
  Copyright : simulink/Model-Wide Utilities/Model Info  Frame=on  DisplayStringWithTags=|  HorizontalTextAlignment=Left  LeftAlignmentValue=0.02
      | © ITK Engineering Technology (Wu Xi) Co., Ltd. (ITKC)
      | 
      | Model Version: %<ModelVersion>
      | Date: %<LastModificationDate>
  InlineDescription : ITKLib/Special/InlineDescription  Tag=HideFromReport  Description=停车检测  ShowInLibBrowser=0  RefreshPar=0
      settings: SourceProductName=ITKC_Lib
  Logical Operator1 : Logic  Operator=OR  Inputs=3  AllPortsSameDT=off  OutDataTypeStr=boolean
  Logical Operator2 : Logic  AllPortsSameDT=off  OutDataTypeStr=boolean
  Logical Operator3 : Logic  Operator=OR  AllPortsSameDT=off  OutDataTypeStr=boolean
  Logical Operator4 : Logic  Operator=OR  Inputs=3  AllPortsSameDT=off  OutDataTypeStr=boolean
  Logical Operator5 : Logic  Operator=NOT  AllPortsSameDT=off  OutDataTypeStr=boolean
  Lower : RelationalOperator  Operator=<  OutDataTypeStr=boolean
  RSLatch : ITKLib/Memory/RSLatch
      settings: SourceProductName=ITKC_Lib
  Relational Operator1 : RelationalOperator  Operator===  OutDataTypeStr=boolean  InputSameDT=off
  Relational Operator3 : RelationalOperator  Operator===  OutDataTypeStr=boolean  InputSameDT=off
  Relational Operator7 : RelationalOperator  Operator===  OutDataTypeStr=boolean  InputSameDT=off
  Switch1 : Switch  Criteria=u2 ~= 0  SaturateOnIntegerOverflow=off  InputSameDT=off
  Switch4 : Switch  Criteria=u2 ~= 0  SaturateOnIntegerOverflow=off  InputSameDT=off
  Unit detailed design : simulink/Model-Wide Utilities/DocBlock  Tag=HideFromReport  DocumentType=Text
      content=|
      | SMiVCU-3260 - 停车运行充放电标志位
      | 同时满足以下条件，则激活[停车运行充放电标志位]
      | 1.<整车电源状态>为0x1：on时：<EPB系统状态>为0x1：Applied或<VCU内部实际挡位状态>为0x4：N或0x6：P
      |    <整车电源状态>不为0x1：on时，以上条件满足时激活并锁存，待[AC充电连接标志位]为0时Reset；
      | 2.<实际车速>小于一定值（HvCoorn_vMax4ChDchgEna_C，2kph）
  dhc_bParkChk4ChDchgMan_C : Constant  Description=[0]  Value=HvCoorn_bParkChk4ChDchgOvrd_C
      settings: AttributesFormatString=%<Description>
  dhc_bParkChk4ChDchgMan_C1 : Constant  Description=[1]  Value=HvCoorn_bParkChk4ChDchgOvrdVal_C
      settings: AttributesFormatString=%<Description>
  hpp_bEpbPark4ChDchgEna_C : Constant  Description=[1]  Value=HvCoorn_bEpbPark4ChDchgEna_C
      settings: AttributesFormatString=%<Description>
  hpp_bEpbPark4ChDchgEna_C1 : Constant  Description=[1]  Value=EPBActSt_Appld_SC
      settings: AttributesFormatString=%<Description>
  hpp_bEpbPark4ChDchgEna_C2 : Constant  Description=[6]  Value=GearLvr_stDrvGearP_SC  OutDataTypeStr=uint8
      settings: AttributesFormatString=%<Description>
  hpp_bEpbPark4ChDchgEna_C3 : Constant  Description=[3]  Value=HvCoorn_vMax4ChDchgEna_C
      settings: AttributesFormatString=%<Description>
  hpp_bEpbPark4ChDchgEna_C4 : Constant  Description=[4]  Value=GearLvr_stDrvGearN_SC  OutDataTypeStr=uint8
      settings: AttributesFormatString=%<Description>
  hpp_bKeyOffParkNoChk_C : Constant  Description=[0]  Value=HvCoorn_bKeyOffParkNoChk_C
      settings: AttributesFormatString=%<Description>
  HvCoorn_bParked4ChDchg : Outport  VectorParamsAs1DForOutWhenUnconnected=off
  wires:
  GearLvr_stDrvGear/1 -> Relational Operator1/1, Relational Operator7/1
  hpp_bEpbPark4ChDchgEna_C2/1 -> Relational Operator7/2
  idi_bKeyOn/1 -> Switch1/2
  dhc_bParkChk4ChDchgMan_C/1 -> Switch4/2
  AND/1 -> Switch4/3  "HvCoorn_bParked4ChDchgRaw"
  HvCoorn_bACChrgLink/1 -> Logical Operator1/1
  Switch4/1 -> HvCoorn_bParked4ChDchg/1
  RSLatch/1 -> Logical Operator3/1
  Logical Operator3/1 -> Switch1/3
  hpp_bKeyOffParkNoChk_C/1 -> Logical Operator3/2
  Logical Operator1/1 -> Logical Operator5/1
  icepb_stEpbSys/1 -> Relational Operator3/1
  hpp_bEpbPark4ChDchgEna_C1/1 -> Relational Operator3/2
  Relational Operator3/1 -> Logical Operator2/1
  hpp_bEpbPark4ChDchgEna_C/1 -> Logical Operator2/2
  Logical Operator2/1 -> Logical Operator4/1
  Relational Operator7/1 -> Logical Operator4/2
  Logical Operator4/1 -> RSLatch/1, Switch1/1  "HvCoorn_bParkedActv"
  dhc_bParkChk4ChDchgMan_C1/1 -> Switch4/1
  VehSpd_vVeh/1 -> Lower/1
  Switch1/1 -> AND/1
  Lower/1 -> AND/2
  hpp_bEpbPark4ChDchgEna_C3/1 -> Lower/2
  hpp_bEpbPark4ChDchgEna_C4/1 -> Relational Operator1/2
  Relational Operator1/1 -> Logical Operator4/3
  HvCoorn_bDCChrgLink/1 -> Logical Operator1/2
  Logical Operator5/1 -> RSLatch/2
  icobc_bDchrgrCnct/1 -> Logical Operator1/3

== system HvCoorn/HvCoorn/HVP_HighVoltagePowerOnOffProcedure/A01_HighvoltPowerUpReq/B05_BattWarmReq ==
  note: This subsystem calculates HV battery warm flag and warm time status.
  icbms_pctHVBatSOCDisp : Inport
  std_tExterTemp : Inport  Port=2
  icbms_bBatACChrgFull : Inport  Port=3
  icacu_stWarmTime : Inport  Port=4
  HvCoorn_bACChrgLink : Inport  Port=5
  iud_bNoHVHConfig : Inport  Port=6
  iud_bNoHVHWarmTiCfg : Inport  Port=7
  inv_stHvBattWarmTime : Inport  Port=8
  DataTypeConversion : DataTypeConversion  OutDataTypeStr=single  SaturateOnIntegerOverflow=off  RndMeth=Floor
  FALSE : Constant  Description=FALSE  Value=0  OutDataTypeStr=boolean
      settings: AttributesFormatString=%<Description>
  Logical Operator{1,3,5,7..8} (5 alike) : Logic  Operator=NOT  Inputs=1  AllPortsSameDT=off  OutDataTypeStr=boolean
  Logical Operator18 : Logic  Inputs=3  AllPortsSameDT=off  OutDataTypeStr=boolean
  Logical Operator2 : Logic  AllPortsSameDT=off  OutDataTypeStr=boolean
  Logical Operator6 : Logic  Inputs=3  AllPortsSameDT=off  OutDataTypeStr=boolean
  Product10 : Product  Inputs=**  RndMeth=Zero  SaturateOnIntegerOverflow=on
  RSLatch : ITKLib/Memory/RSLatch
      settings: SourceProductName=ITKC_Lib
  RSLatch1 : ITKLib/Memory/RSLatch
      settings: SourceProductName=ITKC_Lib
  Relational Operator1 : RelationalOperator  Operator=<=  OutDataTypeStr=boolean  InputSameDT=off
  Relational Operator2 : RelationalOperator  OutDataTypeStr=boolean  InputSameDT=off
  Relational Operator3 : RelationalOperator  OutDataTypeStr=boolean  InputSameDT=off
  Relational Operator4 : RelationalOperator  Operator===  OutDataTypeStr=boolean  InputSameDT=off
  Relational Operator6 : RelationalOperator  OutDataTypeStr=boolean  InputSameDT=off
  Saturation2 : Saturate  UpperLimit=15  LowerLimit=0  OutDataTypeStr=uint8
      settings: AttributesFormatString=<limits=%<UpperLimit>/%<LowerLimit>>
  StopWatchRE : ITKLib/TimeCounter/StopWatchRE  Description=""
      settings: SourceProductName=ITKC_Lib
  Switch : Switch  Criteria=u2 ~= 0  SaturateOnIntegerOverflow=off  InputSameDT=off
      settings: AttributesFormatString=Criteria : %<Criteria>
  Switch1 : Switch  Criteria=u2 ~= 0  SaturateOnIntegerOverflow=off  InputSameDT=off
      settings: AttributesFormatString=Criteria : %<Criteria>
  Switch2 : Switch  Criteria=u2 ~= 0  SaturateOnIntegerOverflow=off  InputSameDT=off
      settings: AttributesFormatString=Criteria : %<Criteria>
  TaskTime_s1 : Constant  Value=TaskTime_10ms
      settings: AttributesFormatString=[0.01]
  TaskTime_s2 : Constant  Value=TaskTime_10ms
      settings: AttributesFormatString=[0.01]
  TurnOnDelayVari : ITKLib/TimeCounter/TurnOnDelayVari
      settings: AttributesFormatString=TurnOnDelay  SourceProductName=ITKC_Lib
  Unit Delay1 : UnitDelay  SampleTime=-1  HasFrameUpgradeWarning=on
      settings: AttributesFormatString=<initial=%<X0>>
  hpp_bWarmTimeConfigEna_C : Constant  Description=[0]  Value=HvCoorn_bWarmTimeCfgEna_C
      settings: AttributesFormatString=%<Description>
  hpp_percBatWarmSocThr_C : Constant  Description=[80]  Value=HvCoorn_pctBatWarmSocThd_C
      settings: AttributesFormatString=%<Description>
  hpp_stDefltWarmTime_C : Constant  Description=[12]  Value=HvCoorn_stDftWarmTime_C
      settings: AttributesFormatString=%<Description>
  hpp_stDefltWarmTime_C1 : Constant  Description=[12]  Value=HvCoorn_stDftWarmTime_C
      settings: AttributesFormatString=%<Description>
  hpp_tBatWarmExterTempThr_C : Constant  Description=[10]  Value=HvCoorn_tBatWarmExterTempThd_C
      settings: AttributesFormatString=%<Description>
  hpp_tiWarmChoseConfirm_C : Constant  Description=[0.05]  Value=HvCoorn_tiWarmChoseCfm_C
      settings: AttributesFormatString=%<Description>
  single : Constant  Value=3600  OutDataTypeStr=single
      settings: AttributesFormatString=%<OutDataTypeStr>
  switch1 : Switch  Criteria=u2 ~= 0  SaturateOnIntegerOverflow=off  InputSameDT=off
  switch2 : Switch  Criteria=u2 ~= 0  OutDataTypeStr=uint8  SaturateOnIntegerOverflow=off  InputSameDT=off
  uint2 : Constant  Description=WarmOff  Value=15  OutDataTypeStr=uint8
      settings: AttributesFormatString=|
      | %<OutDataTypeStr>
      | %<Description>
  uint3 : Constant  Value=0  OutDataTypeStr=uint8
      settings: AttributesFormatString=|
      | %<OutDataTypeStr>
      | %<Description>
  uint8 : Constant  Description=1h  OutDataTypeStr=uint8
      settings: AttributesFormatString=|
      | %<OutDataTypeStr>
      | %<Description>
  HvCoorn_bBattWarmReq : Outport  VectorParamsAs1DForOutWhenUnconnected=off
  HvCoorn_stWarmTimeCfgResp : Outport  Port=2  VectorParamsAs1DForOutWhenUnconnected=off
  wires:
  icbms_pctHVBatSOCDisp/1 -> Relational Operator3/1
  hpp_percBatWarmSocThr_C/1 -> Relational Operator3/2
  Logical Operator6/1 -> RSLatch/1
  hpp_tBatWarmExterTempThr_C/1 -> Relational Operator1/2
  HvCoorn_bACChrgLink/1 -> Logical Operator18/3, Logical Operator7/1, Logical Operator1/1
  Logical Operator18/1 -> StopWatchRE/1, Logical Operator2/1
  Relational Operator6/1 -> Logical Operator8/1
  std_tExterTemp/1 -> Relational Operator1/1
  Logical Operator1/1 -> RSLatch/2
  Logical Operator2/1 -> HvCoorn_bBattWarmReq/1
  StopWatchRE/1 -> Relational Operator6/1
  Logical Operator7/1 -> StopWatchRE/2
  TaskTime_s2/1 -> StopWatchRE/3
  TaskTime_s1/1 -> TurnOnDelayVari/2
  Relational Operator2/1 -> TurnOnDelayVari/1
  hpp_tiWarmChoseConfirm_C/1 -> TurnOnDelayVari/3
  icacu_stWarmTime/1 -> switch1/1, Relational Operator2/1
  uint8/1 -> Relational Operator2/2
  switch1/1 -> Unit Delay1/1, Saturation2/1
  single/1 -> Product10/2
  Product10/1 -> Relational Operator6/2
  Switch/1 -> DataTypeConversion/1
  hpp_bWarmTimeConfigEna_C/1 -> Switch/2
  hpp_stDefltWarmTime_C1/1 -> Switch/1
  RSLatch/1 -> Logical Operator18/2
  Relational Operator3/1 -> Logical Operator6/1
  iud_bNoHVHConfig/1 -> Logical Operator3/1
  Saturation2/1 -> Switch2/3, HvCoorn_stWarmTimeCfgResp/1
  iud_bNoHVHWarmTiCfg/1 -> Switch2/2
  hpp_stDefltWarmTime_C/1 -> Switch2/1
  Switch2/1 -> Switch1/3, Relational Operator4/1
  uint2/1 -> Relational Operator4/2
  Relational Operator4/1 -> Switch1/2
  uint3/1 -> Switch1/1
  Switch1/1 -> Switch/3
  Relational Operator1/1 -> Logical Operator6/3
  icbms_bBatACChrgFull/1 -> Logical Operator6/2
  Logical Operator8/1 -> Logical Operator2/2
  Unit Delay1/1 -> switch2/3
  Logical Operator5/1 -> switch2/2
  TurnOnDelayVari/1 -> RSLatch1/1, switch1/2
  RSLatch1/1 -> Logical Operator5/1
  inv_stHvBattWarmTime/1 -> switch2/1
  FALSE/1 -> RSLatch1/2
  switch2/1 -> switch1/3
  DataTypeConversion/1 -> Product10/1
  Logical Operator3/1 -> Logical Operator18/1

== system HvCoorn/HvCoorn/HVP_HighVoltagePowerOnOffProcedure/A01_HighvoltPowerUpReq/B06_ChgrCnctStCal ==
  note: This subsystem calculates AC Charger link flag, AC Charger link OK flag and AC Charger link pause flag, based on CC status, CP flag, CP voltage and vehicle velocity .
  note: Documentation
  HvCoorn_bObcChrgrCnct : Inport
  icobc_bChrgrCtrlSigCnct : Inport  Port=2
  icobc_uChrgrCtrlSigVolt : Inport  Port=3
  VehSpd_vVeh : Inport  Port=4
  icbms_stDcChrgrCnct : Inport  Port=5
  icobc_bDchrgrCnct : Inport  Port=6
  icobc_bVehCnct : Inport  Port=7
  AND : Logic  OutDataTypeStr=boolean
  Abs1 : Abs
  Copyright : simulink/Model-Wide Utilities/Model Info  Frame=on  DisplayStringWithTags=|  HorizontalTextAlignment=Left  LeftAlignmentValue=0.02
      | © ITK Engineering Technology (Wu Xi) Co., Ltd. (ITKC)
      | 
      | Model Version: %<ModelVersion>
      | Date: %<LastModificationDate>
  InlineDescription : ITKLib/Special/InlineDescription  Tag=HideFromReport  Description=充电连接状态确认  ShowInLibBrowser=0  RefreshPar=0
      settings: SourceProductName=ITKC_Lib
  Logical Operator1 : Logic  Operator=OR  Inputs=3  AllPortsSameDT=off  OutDataTypeStr=boolean
  Logical Operator14 : Logic  Operator=NOT  Inputs=1  AllPortsSameDT=off  OutDataTypeStr=boolean
  Logical Operator{2,5,16..17} (4 alike) : Logic  AllPortsSameDT=off  OutDataTypeStr=boolean
  Logical Operator3 : Logic  Inputs=3  AllPortsSameDT=off  OutDataTypeStr=boolean
  Logical Operator7 : Logic  Inputs=3  AllPortsSameDT=off  OutDataTypeStr=boolean
  Logical Operator8 : Logic  Operator=OR  Inputs=3  AllPortsSameDT=off  OutDataTypeStr=boolean
  Logical Operator9 : Logic  Operator=OR  AllPortsSameDT=off  OutDataTypeStr=boolean
  Not : Logic  Operator=NOT  AllPortsSameDT=off  OutDataTypeStr=boolean
  OR : Logic  Operator=OR  OutDataTypeStr=boolean
  OR1 : Logic  Operator=OR  OutDataTypeStr=boolean
  Relational Operator1 : RelationalOperator  Operator=<=  OutDataTypeStr=boolean  InputSameDT=off
  Relational Operator5 : RelationalOperator  Operator===  OutDataTypeStr=boolean  InputSameDT=off
  Relational Operator6 : RelationalOperator  OutDataTypeStr=boolean  InputSameDT=off
  Relational Operator9 : RelationalOperator  Operator===  OutDataTypeStr=boolean  InputSameDT=off
  TaskTime_s1 : Constant  Value=TaskTime_10ms
      settings: AttributesFormatString=[0.01]
  TaskTime_s2 : Constant  Value=TaskTime_10ms
      settings: AttributesFormatString=[0.01]
  TurnOnDelayVari : ITKLib/TimeCounter/TurnOnDelayVari
      settings: AttributesFormatString=TurnOnDelay  SourceProductName=ITKC_Lib
  TurnOnDelayVari1 : ITKLib/TimeCounter/TurnOnDelayVari
      settings: AttributesFormatString=TurnOnDelay  SourceProductName=ITKC_Lib
  Unit detailed design : simulink/Model-Wide Utilities/DocBlock  Tag=HideFromReport  DocumentType=Text
      content=|
      | SMiVCU-3275 - DC充电连接标志位
      | 同时满足以下条件，则激活[DC充电连接标志位]：
      | 1.<DC充电连接状态>为0x1：WakeupInactive，或0x2：WakeupActive；
      | 2.<实际车速>小于一定值（HvCoorn_vVldChrgLinkThd_C，初始值1.5kph）。
      |
      | SMiVCU-3276 - AC充电连接标志位
      | 同时满足以下条件，则激活[AC充电连接标志位]：
      | 1.<实际车速>小于一定值（HvCoorn_vVldChrgLinkThd_C，初始值1.5kph）。
      | 2.<充电激活输出状态>为1，或<OBC充电连接状态>为0x1：Half Connect或0x2：Connected或0x3：V2VConnected或0x4：V2LConnected。
      |
      | SMiVCU-3277 - 充电枪连接标志位
      | [DC充电连接标志位]或[AC充电连接标志位]为1，则激活[充电枪连接标志位]。
      |
      | SMiVCU-3274 - AC充电暂停标志位
      | 以下条件同时满足，则激活[AC充电暂停标志位]：
      | 1.[AC充电连接标志位]为1；
      | 2.[OBC充电连接状态]不为0x3：V2VConnected或0x4：V2LConnected；
      | 3.[OBC充电连接状态]不为0x2：Connected或<充电激活输出状态>不为1；
  hpp_tiCpConnectCheck_C : Constant  Description=[0.1]  Value=HvCoorn_tiCpConnectChk_C
      settings: AttributesFormatString=%<Description>
  hpp_tiSpdVld4ChgLinkChk_C : Constant  Description=[0.1]  Value=HvCoorn_tiSpdVld4ChrgLinkChk_C
      settings: AttributesFormatString=%<Description>
  hpp_tiSpdVld4ChgLinkChk_C1 : Constant  Description=[1]  Value=HvCoorn_bDCChrgFctCfg_C
      settings: AttributesFormatString=%<Description>
  hpp_tiSpdVld4ChgLinkChk_C2 : Constant  Description=[1]  Value=HvCoorn_bDcChrgWkupEnaChrgLink_C
      settings: AttributesFormatString=%<Description>
  hpp_tiSpdVld4ChgLinkChk_C3 : Constant  Description=[0]  Value=HvCoorn_bDCDcnct4ACEna_C
      settings: AttributesFormatString=%<Description>
  hpp_uCpConnectCheck_C : Constant  Description=[1000]  Value=HvCoorn_uCpConnectChk_C
      settings: AttributesFormatString=%<Description>
  hpp_vVldChgLinkThr_C : Constant  Description=[3]  Value=HvCoorn_vVldChrgLinkThd_C
      settings: AttributesFormatString=%<Description>
  uint5 : Constant  Description=DCPlug_WakeupInactive  OutDataTypeStr=uint8
      settings: AttributesFormatString=|
      | %<OutDataTypeStr>
      | %<Description>
  uint6 : Constant  Description=DCPlug_WakeupActive  Value=2  OutDataTypeStr=uint8
      settings: AttributesFormatString=|
      | %<OutDataTypeStr>
      | %<Description>
  HvCoorn_bACChrgLinkOk : Outport  VectorParamsAs1DForOutWhenUnconnected=off
  HvCoorn_bACChrgLink : Outport  Port=2  VectorParamsAs1DForOutWhenUnconnected=off
  HvCoorn_bACChrgPause : Outport  Port=3  VectorParamsAs1DForOutWhenUnconnected=off
  HvCoorn_bDCChrgLink : Outport  Port=4  VectorParamsAs1DForOutWhenUnconnected=off
  HvCoorn_bChrgLink : Outport  Port=5  VectorParamsAs1DForOutWhenUnconnected=off
  wires:
  OR/1 -> Logical Operator17/1, Logical Operator1/3
  icobc_uChrgrCtrlSigVolt/1 -> Relational Operator6/1
  hpp_uCpConnectCheck_C/1 -> Relational Operator6/2
  Relational Operator6/1 -> TurnOnDelayVari1/1
  Logical Operator16/1 -> HvCoorn_bACChrgPause/1
  Logical Operator14/1 -> Logical Operator16/2
  TurnOnDelayVari1/1 -> Logical Operator1/1
  icobc_bChrgrCtrlSigCnct/1 -> Logical Operator17/2, Logical Operator1/2
  Logical Operator17/1 -> Logical Operator14/1, Logical Operator5/2
  VehSpd_vVeh/1 -> Abs1/1
  Logical Operator3/1 -> Logical Operator16/1, HvCoorn_bACChrgLink/1, Logical Operator8/3, [HvCoorn_bACChrgLink]
  Logical Operator5/1 -> HvCoorn_bACChrgLinkOk/1
  hpp_vVldChgLinkThr_C/1 -> Relational Operator1/2
  Abs1/1 -> Relational Operator1/1
  Logical Operator1/1 -> Logical Operator3/2  "ACChgLinkRaw"
  TurnOnDelayVari/1 -> [HvCoorn_bVehVLow], Logical Operator3/1
  hpp_tiCpConnectCheck_C/1 -> TurnOnDelayVari1/3
  hpp_tiSpdVld4ChgLinkChk_C/1 -> TurnOnDelayVari/3
  TaskTime_s2/1 -> TurnOnDelayVari/2
  Relational Operator1/1 -> TurnOnDelayVari/1
  [HvCoorn_bACChrgLink] -> Logical Operator5/1
  TaskTime_s1/1 -> TurnOnDelayVari1/2
  Relational Operator9/1 -> AND/1
  icbms_stDcChrgrCnct/1 -> Relational Operator5/1, Relational Operator9/1
  Relational Operator5/1 -> [HvCoorn_bDCChrgWkup], Logical Operator9/2
  Logical Operator9/1 -> Logical Operator7/1
  hpp_tiSpdVld4ChgLinkChk_C1/1 -> Logical Operator7/3
  [HvCoorn_bVehVLow] -> Logical Operator7/2
  Logical Operator7/1 -> Logical Operator8/1, HvCoorn_bDCChrgLink/1
  Logical Operator8/1 -> HvCoorn_bChrgLink/1
  uint5/1 -> Relational Operator9/2
  uint6/1 -> Relational Operator5/2
  AND/1 -> Logical Operator9/1
  hpp_tiSpdVld4ChgLinkChk_C2/1 -> AND/2
  Logical Operator2/1 -> Logical Operator8/2
  icobc_bDchrgrCnct/1 -> Logical Operator2/1
  [HvCoorn_bVehVLow] -> Logical Operator2/2
  icobc_bVehCnct/1 -> OR/2
  HvCoorn_bObcChrgrCnct/1 -> OR/1
  [HvCoorn_bDCChrgWkup] -> Not/1
  hpp_tiSpdVld4ChgLinkChk_C3/1 -> OR1/2
  Not/1 -> OR1/1
  OR1/1 -> Logical Operator3/3
